simulink model "G13_sim"  (R2024b)
settings: Solver=VariableStepAuto  StartTime=0.0  StopTime=10.0  RelTol=1e-3
values from neighbouring files (symbols this model uses):
  Cdc = 2*Pdc/(fac*(((1+DeltaUdc/2)*Udc)^2-((1-DeltaUdc/2)*Udc)^2))    (= 0.204081632653)    [AC_DC_G13.m]
  fac = 50    [AC_DC_G13.m]
  Lfac = Udc/(6*fpwm_inv*DeltaIac)    (= 0.000809045226131)    [AC_DC_G13.m]
  Pac = 200e3/3    (= 66666.6666667)    [AC_DC_G13.m]
  QCac = QLac-(Pac*tan(acos(Fp)))    [AC_DC_G13.m]
  QLac = Pac*tan(acos(Fpi))    [AC_DC_G13.m]
  Rdc = Udc^2/(Pdc-Pdcmin)    (= 5.44444444444)    [AC_DC_G13.m]
  Rdcmax = Udc^2/Pdcmin    (= 49)    [AC_DC_G13.m]
  Udc = 700    [AC_DC_G13.m]
  Vac = 230    [AC_DC_G13.m]
  Vdcref = Udc    (= 700)    [AC_DC_G13.m]
undefined symbols (not defined in the file or in its folder): fpwm
libraries: spsSeriesRLCBranchLib x6, spsThreePhaseVIMeasurementLib x3, spsCurrentMeasurementLib x2, spsIdealSwitchLib x1, eePowerMeasurement x1, spsMeanLib x1, spsThreePhaseHarmonicFilterLib x1, spsThreePhaseParallelRLCLoadLib x1, spsThreePhaseSourceLib x1, spsUniversalBridgeLib x1, spsVoltageMeasurementLib x1
settings Model: Creator=franc  LastModifiedBy=franc

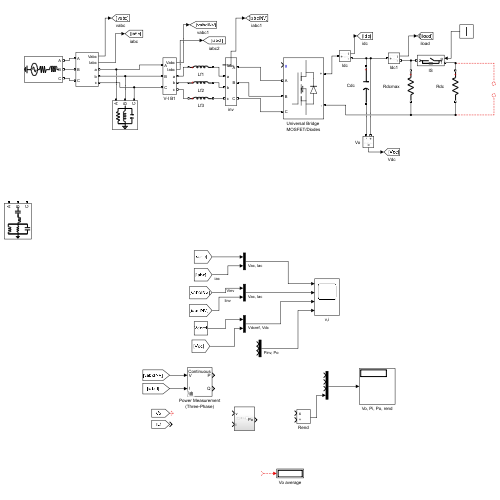
[thumbnail: Simulink's stored preview of the top-level diagram]
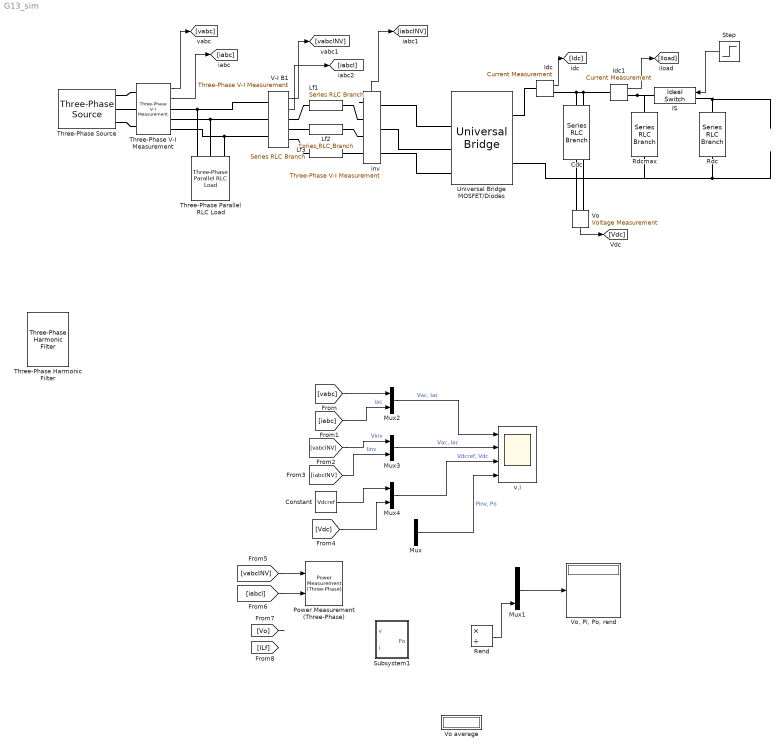
== system G13_sim ==
  Cdc : spsSeriesRLCBranchLib/Series RLC Branch  LConnTagsString=__new0  RConnTagsString=__new0  BranchType=C  Resistance=1  Inductance=1e-3  SetiL0=off  InitialCurrent=0  Capacitance=Cdc  Setx0=on  InitialVoltage=0.75*Udc  Measurements=None
  Constant : Constant  Value=Vdcref
  IS : spsIdealSwitchLib/Ideal Switch  Ron=0.001  Lon=0  IC=0  Rs=1e5  Cs=inf  Measurements=off
  Idc : spsCurrentMeasurementLib/Current Measurement  PhasorSimulation=off  OutputType=Complex  PSBequivalent=0
  Idc1 : spsCurrentMeasurementLib/Current Measurement  PhasorSimulation=off  OutputType=Complex  PSBequivalent=0
  Lf1 : spsSeriesRLCBranchLib/Series RLC Branch  LConnTagsString=__new0  RConnTagsString=__new0  BranchType=L  Resistance=1  Inductance=Lfac  SetiL0=off  InitialCurrent=0  Capacitance=1e-6  Setx0=off  InitialVoltage=0  Measurements=None
  Lf2 : spsSeriesRLCBranchLib/Series RLC Branch  LConnTagsString=__new0  RConnTagsString=__new0  BranchType=L  Resistance=1  Inductance=Lfac  SetiL0=off  InitialCurrent=0  Capacitance=1e-6  Setx0=off  InitialVoltage=0  Measurements=None
  Lf3 : spsSeriesRLCBranchLib/Series RLC Branch  LConnTagsString=__new0  RConnTagsString=__new0  BranchType=L  Resistance=1  Inductance=Lfac  SetiL0=off  InitialCurrent=0  Capacitance=1e-6  Setx0=off  InitialVoltage=0  Measurements=None
  Mux : Mux  Inputs=3
  Mux1 : Mux
  Mux2 : Mux  Inputs=2
  Mux3 : Mux  Inputs=2
  Mux4 : Mux  Inputs=2
  Power Measurement (Three-Phase) : eePowerMeasurement/Power Measurement (Three-Phase)  LabelModeActiveChoice=Continuous  F=60  K=[0 1 2 3]  Seq=Positive  Ts=0
  Rdc : spsSeriesRLCBranchLib/Series RLC Branch  LConnTagsString=__new0  RConnTagsString=__new0  BranchType=R  Resistance=Rdc  Inductance=1e-3  SetiL0=off  InitialCurrent=0  Capacitance=1e-6  Setx0=off  InitialVoltage=0  Measurements=None
  Rdcmax : spsSeriesRLCBranchLib/Series RLC Branch  LConnTagsString=__new0  RConnTagsString=__new0  BranchType=R  Resistance=Rdcmax  Inductance=1e-3  SetiL0=off  InitialCurrent=0  Capacitance=1e-6  Setx0=off  InitialVoltage=0  Measurements=None
  Rend : Product  Inputs=*/
  Step : Step  Time=0.06  SampleTime=0
  Subsystem1 : Subsystem
  Three-Phase Harmonic Filter : spsThreePhaseHarmonicFilterLib/Three-Phase Harmonic Filter  LConnTagsString=A|B|C  FilterType=Double-tuned  FilterConnection=Y (grounded)  ParNom=[315e3 60]  Qc=49e6  Fr=[5*60]  Frd=[11*60 13*60]  Q=16  Measurements=None
      settings: AttributesFormatString=\n
      settings: LibrarySourceBlock=|
      | sps_lib/Passives/Three-Phase
      | Harmonic Filter
  Three-Phase Parallel RLC Load : spsThreePhaseParallelRLCLoadLib/Three-Phase Parallel RLC Load  LConnTagsString=A|B|C  Configuration=Y (grounded)  NominalVoltage=Vac*sqrt(3)  Vabc=[1e3 1e3 1e3]  Vabcp=[1e3 1e3 1e3]  NominalFrequency=fac  UnbalancedPower=off  ActivePower=Pac*3  InductivePower=QLac*3  CapacitivePower=QCac*3  Pabc=[10e3 9e3 11e3]  QLabc=[100 90 110]  QCabc=[100 90 110]  Pabcp=[10e3 9e3 11e3]  QLabcp=[100 90 110]  QCabcp=[100 90 110]  Measurements=None  LoadType=constant Z
  Three-Phase V-I Measurement : spsThreePhaseVIMeasurementLib/Three-Phase V-I Measurement  VoltageMeasurement=phase-to-ground  SetLabelV=off  LabelV=Vabc  Vpu=off  VpuLL=off  CurrentMeasurement=yes  SetLabelI=off  LabelI=Iabc  Ipu=off  Pbase=100e6  Vbase=500e3  OutputType=Complex  PhasorSimulation=off  PSBequivalent=0
  Three-Phase Source : spsThreePhaseSourceLib/Three-Phase Source  InternalConnection=Yg  VoltagePhases=off  Voltage=Vac*sqrt(3)  PhaseAngle=0  Voltage_phases=[25e3 25e3 25e3]/sqrt(3)  PhaseAngles_phases=[0 -120 +120]  Frequency=fac  NonIdealSource=on  SpecifyImpedance=on  Resistance=0.8929  Inductance=16.58e-3  ShortCircuitLevel=Scc  BaseVoltage=Vac*sqrt(3)  XRratio=X_R  BusType=swing  Pref=10e3  Qref=0  Prefabc=[10e3, 10e3, 10e3]  Qrefabc=[0, 0, 0]  Qmin=-inf  Qmax=inf
  Universal Bridge MOSFET/Diodes : spsUniversalBridgeLib/Universal Bridge  Arms=3  SnubberResistance=Rs  SnubberCapacitance=inf  Device=MOSFET / Diodes  Ron=Ron  Lon=0  ForwardVoltages="[  0  0  ]"  ForwardVoltage=0  GTOparameters=[ 10e-6 , 20e-6 ]  IGBTparameters=[ 1e-6 , 2e-6 ]  Measurements=None  Measurements_2=None  converterType=Rectifier
  V-I B1 : spsThreePhaseVIMeasurementLib/Three-Phase V-I Measurement  VoltageMeasurement=phase-to-ground  SetLabelV=off  LabelV=Vabc  Vpu=off  VpuLL=off  CurrentMeasurement=yes  SetLabelI=off  LabelI=Iabc  Ipu=off  Pbase=100e6  Vbase=500e3  OutputType=Complex  PhasorSimulation=off  PSBequivalent=0
  Vo : spsVoltageMeasurementLib/Voltage Measurement  PhasorSimulation=off  OutputType=Complex  PSBequivalent=0
  Vo average : Display
  "Vo, Pi, Po, rend" : Display
  inv : spsThreePhaseVIMeasurementLib/Three-Phase V-I Measurement  VoltageMeasurement=no  SetLabelV=off  LabelV=Vabc  Vpu=off  VpuLL=off  CurrentMeasurement=yes  SetLabelI=off  LabelI=Iabc  Ipu=off  Pbase=100e6  Vbase=500e3  OutputType=Complex  PhasorSimulation=off  PSBequivalent=0
  v,i : Scope  NumInputPorts=4
  wires:
  Three-Phase V-I Measurement/1 -> [vabc]
  Three-Phase V-I Measurement/2 -> [iabc]
  V-I B1/1 -> [vabcINV]
  V-I B1/2 -> [iabcl]
  inv/1 -> [iabcINV]
  Vo/1 -> [Vdc]
  Idc/1 -> [Idc]
  Idc1/1 -> [Iload]
  Step/1 -> IS/1
  Rend/1 -> Mux1/4
  [Vo] -> ?
  ? -> Vo average/1
  Mux1/1 -> "Vo, Pi, Po, rend"/1
  [iabc] -> Mux2/2  "iac"
  [vabc] -> Mux2/1
  Mux2/1 -> v,i/1  "Vac, Iac"
  [vabcINV] -> Mux3/1  "Vinv"
  [iabcINV] -> Mux3/2  "Iinv"
  Mux3/1 -> v,i/2  "Vac, Iac"
  Constant/1 -> Mux4/1
  [Vdc] -> Mux4/2
  Mux4/1 -> v,i/3  "Vdcref, Vdc"
  Mux/1 -> v,i/4  "Pinv, Po"
  [iabcl] -> Power Measurement (Three-Phase)/2
  [vabcINV] -> Power Measurement (Three-Phase)/1
  connections:
  Three-Phase Source/RConn1 -- Three-Phase V-I Measurement/LConn1
  Three-Phase Source/RConn2 -- Three-Phase V-I Measurement/LConn2
  Three-Phase Source/RConn3 -- Three-Phase V-I Measurement/LConn3
  Three-Phase V-I Measurement/RConn1 -- Three-Phase Parallel RLC Load/LConn1 -- V-I B1/LConn1
  Three-Phase V-I Measurement/RConn2 -- Three-Phase Parallel RLC Load/LConn2 -- V-I B1/LConn2
  Three-Phase V-I Measurement/RConn3 -- Three-Phase Parallel RLC Load/LConn3 -- V-I B1/LConn3
  V-I B1/RConn3 -- Lf3/LConn1
  V-I B1/RConn2 -- Lf2/LConn1
  V-I B1/RConn1 -- Lf1/LConn1
  Vo/LConn2 -- Cdc/RConn1
  Universal Bridge MOSFET/Diodes/RConn1 -- Idc/LConn1
  Idc/RConn1 -- Idc1/LConn1 -- Vo/LConn1 -- Cdc/LConn1
  Idc1/RConn1 -- IS/RConn1 -- Rdcmax/LConn1
  Rdc/LConn1 -- IS/LConn1
  Rdc/RConn1 -- Universal Bridge MOSFET/Diodes/RConn2 -- Rdcmax/RConn1
  inv/LConn1 -- Universal Bridge MOSFET/Diodes/LConn1
  inv/LConn2 -- Universal Bridge MOSFET/Diodes/LConn2
  inv/LConn3 -- Universal Bridge MOSFET/Diodes/LConn3
  Lf3/RConn1 -- inv/RConn3
  Lf2/RConn1 -- inv/RConn2
  Lf1/RConn1 -- inv/RConn1

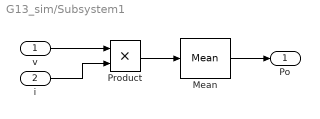
== system G13_sim/Subsystem1 ==
  v : Inport
  i : Inport  Port=2
  Mean : spsMeanLib/Mean  Freq=fpwm/10  Vinit=110  Ts=0
  Product : Product
  Po : Outport
  wires:
  Mean/1 -> Po/1
  i/1 -> Product/2
  v/1 -> Product/1
  Product/1 -> Mean/1
